simulink model "Gravity_Dynamics_Model"  (R2024a)
settings: Solver=VariableStepAuto  StartTime=0.0  StopTime=10.0  RelTol=1e-3
undefined symbols (not defined in the file): g, nu_b_0, p_b_i_0, q_0, UAV
settings Model: Creator=Usuario  LastModifiedBy=Usuario

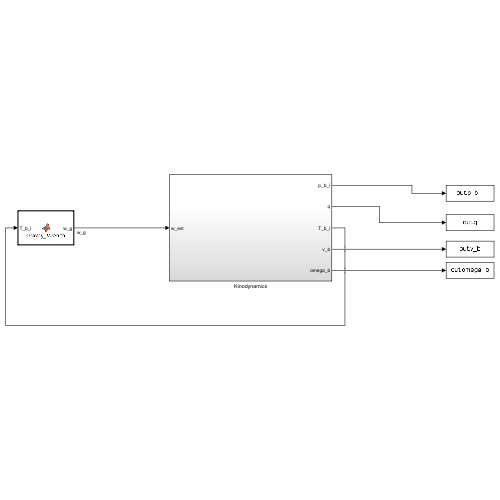
[thumbnail: Simulink's stored preview of the top-level diagram]
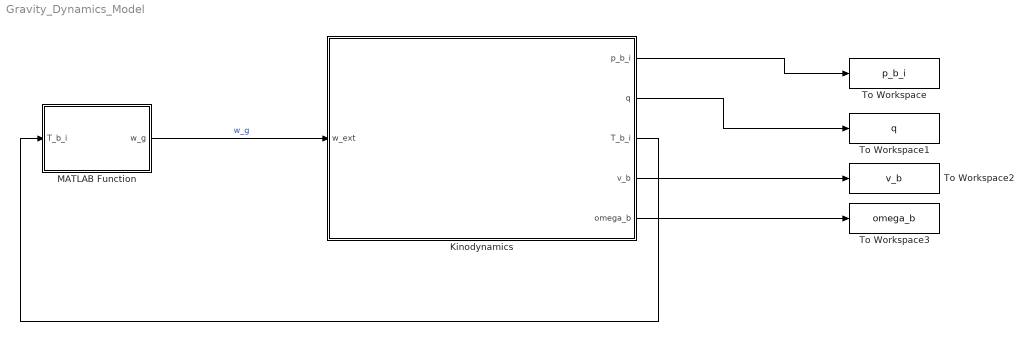
== system Gravity_Dynamics_Model ==
  Kinodynamics : Subsystem
  MATLAB Function : MATLAB Function  TreatAsAtomicUnit=on
  To Workspace : ToWorkspace  VariableName=p_b_i  SaveFormat=Timeseries  SampleTime=-1
  To Workspace1 : ToWorkspace  VariableName=q  SaveFormat=Timeseries  SampleTime=-1
  To Workspace2 : ToWorkspace  VariableName=v_b  SaveFormat=Timeseries  SampleTime=-1
  To Workspace3 : ToWorkspace  VariableName=omega_b  SaveFormat=Timeseries  SampleTime=-1
  wires:
  MATLAB Function/1(w_g) -> Kinodynamics/1(w_ext)  "w_g"
  Kinodynamics/1(p_b_i) -> To Workspace/1
  Kinodynamics/2(q) -> To Workspace1/1
  Kinodynamics/3(T_b_i) -> MATLAB Function/1(T_b_i)
  Kinodynamics/4(v_b) -> To Workspace2/1
  Kinodynamics/5(omega_b) -> To Workspace3/1

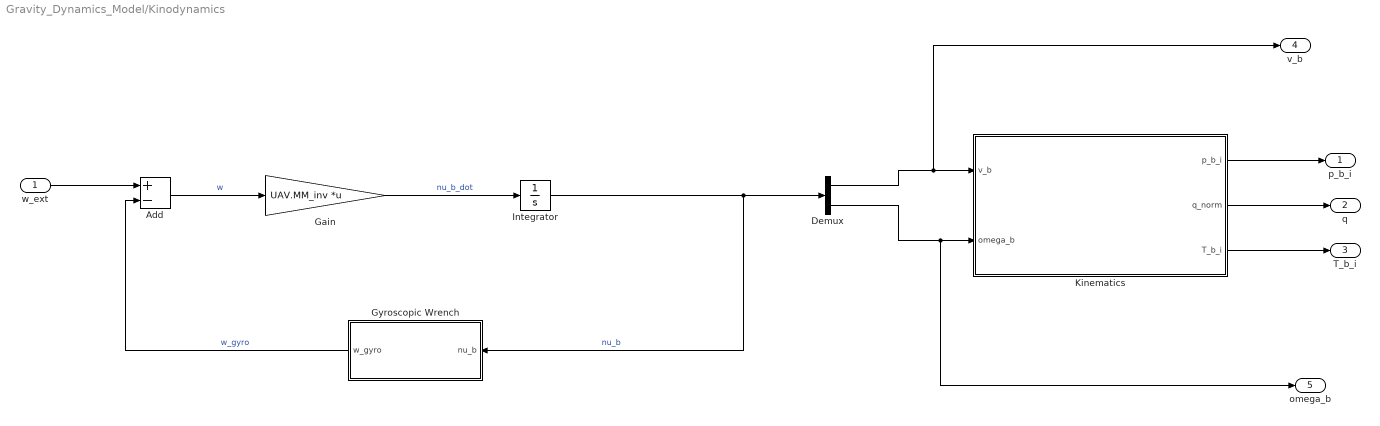
== system Gravity_Dynamics_Model/Kinodynamics ==
  w_ext : Inport
  Add : Sum  Inputs=+-
  Demux : Demux  Outputs=[3 3]
  Gain : Gain  Gain=UAV.MM_inv  Multiplication=Matrix(K*u)
  Gyroscopic Wrench : MATLAB Function  TreatAsAtomicUnit=on
  Integrator : Integrator  InitialCondition=nu_b_0
  Kinematics : Subsystem
  p_b_i : Outport
  q : Outport  Port=2
  T_b_i : Outport  Port=3
  v_b : Outport  Port=4
  omega_b : Outport  Port=5
  wires:
  Kinematics/1(p_b_i) -> p_b_i/1
  w_ext/1 -> Add/1
  Integrator/1 -> Gyroscopic Wrench/1(nu_b), Demux/1  "nu_b"
  Gain/1 -> Integrator/1  "nu_b_dot"
  Demux/2 -> omega_b/1, Kinematics/2(omega_b)
  Kinematics/3(T_b_i) -> T_b_i/1
  Demux/1 -> v_b/1, Kinematics/1(v_b)
  Kinematics/2(q_norm) -> q/1
  Gyroscopic Wrench/1(w_gyro) -> Add/2  "w_gyro"
  Add/1 -> Gain/1  "w"

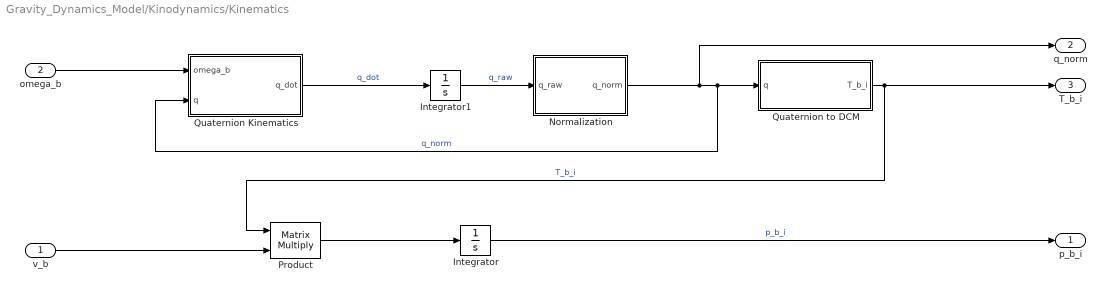
== system Gravity_Dynamics_Model/Kinodynamics/Kinematics ==
  v_b : Inport
  omega_b : Inport  Port=2
  " Normalization" : MATLAB Function  TreatAsAtomicUnit=on
  Integrator : Integrator  InitialCondition=p_b_i_0
  Integrator1 : Integrator  InitialCondition=q_0
  Product : Product  Multiplication=Matrix(*)
  Quaternion Kinematics : MATLAB Function  TreatAsAtomicUnit=on
  Quaternion to DCM : MATLAB Function  TreatAsAtomicUnit=on
  p_b_i : Outport
  q_norm : Outport  Port=2
  T_b_i : Outport  Port=3
  wires:
  Integrator1/1 -> " Normalization"/1(q_raw)  "q_raw"
  " Normalization"/1(q_norm) -> q_norm/1, Quaternion Kinematics/2(q), Quaternion to DCM/1(q)  "q_norm"
  omega_b/1 -> Quaternion Kinematics/1(omega_b)
  Quaternion Kinematics/1(q_dot) -> Integrator1/1  "q_dot"
  Product/1 -> Integrator/1
  Quaternion to DCM/1(T_b_i) -> T_b_i/1, Product/1  "T_b_i"
  v_b/1 -> Product/2
  Integrator/1 -> p_b_i/1  "p_b_i"

== matlab function Gravity_Dynamics_Model/Kinodynamics/Kinematics/ Normalization ==
  data: q_raw input; q_norm output
function q_norm=normalization(q_raw)

q_norm=q_raw/norm(q_raw);

== matlab function Gravity_Dynamics_Model/Kinodynamics/Kinematics/Quaternion Kinematics ==
  data: omega_b input; q_dot output; q input
function q_dot = quat_kinematics(omega_b,q)
%Quaternion kinematics. Requires that omega_b be a column vector. q must
%also be a column vector following the course's quaternion convention. 
eta=q(1);
epsilon=q(2:4);
epsilon_x=cross_matrix(epsilon);

q_dot=1/2*[-epsilon';epsilon_x+eta*eye(3,3)]*omega_b;
end

== matlab function Gravity_Dynamics_Model/Kinodynamics/Gyroscopic Wrench ==
  data: nu_b input; w_gyro output; UAV parameter
function w_gyro=gyroscopic_wrench(nu_b,UAV)
nu_b_southwest=[cross_matrix(nu_b(4:6)),zeros(3,3);cross_matrix(nu_b(1:3)),cross_matrix(nu_b(4:6))];
w_gyro=nu_b_southwest*UAV.MM*nu_b;
end

== matlab function Gravity_Dynamics_Model/MATLAB Function ==
  data: T_b_i input; w_g output; UAV parameter; g parameter
function w_g=Gravity_Wrench(T_b_i,UAV, g)
e3=[0;0;1];

w_g=-g*[UAV.m*T_b_i'*e3;UAV.S*T_b_i'*e3];
end

== matlab function Gravity_Dynamics_Model/Kinodynamics/Kinematics/Quaternion to DCM ==
  data: q input; T_b_i output
function T_b_i=quaternion_to_DCM(q)
%My implementation of the quaternion to DCM transformation, to ensure
%consistency. It must return the active representation of the rotation
%between i and b, which will be the DCM from b to i. 
eta=q(1);
epsilon=q(2:4);
epsilon_x=cross_matrix(epsilon);

T_b_i=eye(3,3)+2*eta*epsilon_x+2*epsilon_x*epsilon_x;
end
